simulink model "fuzzy_BB"  (R2020b)
settings: Solver=FixedStepAuto  StartTime=0.0  StopTime=10.0  FixedStep=0.01  RelTol=1e-3
libraries: fuzblock x1
settings Model: Creator=ACER  LastModifiedBy=ACER

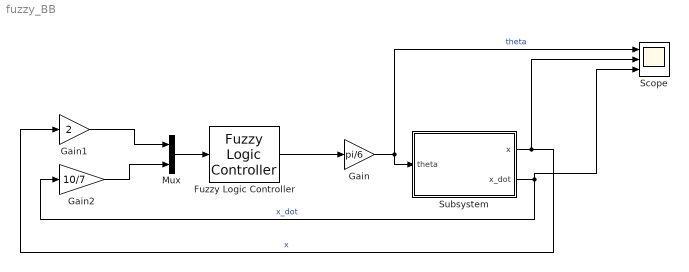
== system fuzzy_BB ==
  Fuzzy Logic Controller : fuzblock/Fuzzy Logic  Controller  FIS='ballandbeam.fis'  OutputSampleNumber=101  DataType=double  FuzzifiedInputs=off  RuleFiringStrengths=off  RuleOutputs=off  AggregatedOutputs=off  SimulateUsing=Interpreted execution  OutOfRangeInputValueMessage=warning  NoRuleFiredMessage=warning  EmptyOutputFuzzySetMessage=warning
  Gain : Gain  Gain=pi/6
  Gain1 : Gain  Gain=2
  Gain2 : Gain  Gain=10/7
  Mux : Mux  Inputs=2
  Scope : Scope  NumInputPorts=3
  Subsystem : Subsystem  mask{x0=-0.25}
  wires:
  Gain1/1 -> Mux/1
  Gain2/1 -> Mux/2
  Mux/1 -> Fuzzy Logic Controller/1
  Fuzzy Logic Controller/1 -> Gain/1
  Gain/1 -> Scope/1, Subsystem/1(theta)  "theta"
  Subsystem/1(x) -> Scope/2, Gain1/1  "x"
  Subsystem/2(x_dot) -> Scope/3, Gain2/1  "x_dot"

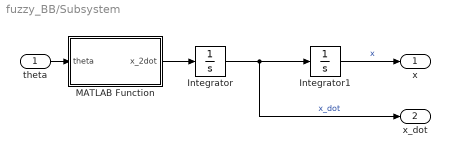
== system fuzzy_BB/Subsystem ==
  theta : Inport
  Integrator : Integrator
  Integrator1 : Integrator  InitialCondition=x0
  MATLAB Function : MATLAB Function  TreatAsAtomicUnit=on
  x : Outport
  x_dot : Outport  Port=2
  wires:
  MATLAB Function/1(x_2dot) -> Integrator/1
  Integrator1/1 -> x/1  "x"
  Integrator/1 -> x_dot/1, Integrator1/1  "x_dot"
  theta/1 -> MATLAB Function/1(theta)

== matlab function fuzzy_BB/Subsystem/MATLAB Function ==
  data: theta input; x_2dot output
function x_2dot = fcn(theta)
%% model parameters
m= 1.7;
R = 5e-3;
J = 3.3e-5;
g= 9.81;
%%
x_2dot = m*g*sin(theta) / (J/R^2 +m)
